simulink model "single2int"  (Simulink 7.6)
settings: Solver=FixedStepDiscrete  StartTime=0.0  StopTime=10000  FixedStep=1  RelTol=1e-3
settings Model: Creator=jordan  LastModifiedBy=jordan
settings DataIOCC: LimitDataPoints=off  SaveOutput=off  SignalLogging=off  DSMLogging=off  SaveTime=off
settings OptimizationCC: BlockReduction=off  ConditionallyExecuteInputs=off

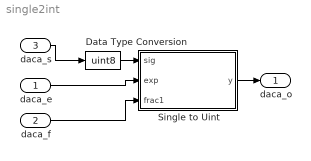
== system single2int ==
  daca_e : Inport  OutDataTypeStr=uint8
  daca_f : Inport  Port=2  OutDataTypeStr=fixdt(0,24,0)
  daca_s : Inport  Port=3  OutDataTypeStr=boolean
  Data Type Conversion : DataTypeConversion  OutDataTypeStr=uint8
  Single to Uint : Stateflow chart  TreatAsAtomicUnit=on
  daca_o : Outport  OutDataTypeStr=fixdt(0,12,0)
  wires:
  Single to Uint/1(y) -> daca_o/1
  daca_e/1 -> Single to Uint/2(exp)
  daca_f/1 -> Single to Uint/3(frac1)
  daca_s/1 -> Data Type Conversion/1
  Data Type Conversion/1 -> Single to Uint/1(sig)

== matlab function Single to Uint ==
  data: sig input uint8; y output fixdt(0,12,0); exp input uint8; frac1 input fixdt(0,24,0)
function y = fcn(sig, exp, frac1)
%#eml

y=fi(0,0,12,0);
z=int16(0);
if (sig==0)
    if (exp>=127)
        buf=uint32(frac1);
        z=int16(exp)-150;
        y=fi(bitshift(buf,z),0,12,0); %-23+(exp-127)
    end
end
